simulink model "Missile"  (R2020a)
settings: Solver=VariableStepAuto  StartTime=0.0  StopTime=inf  RelTol=1e-3
InitFcn:
  | initKRPC
libraries: aerolibutil x2
settings Model: Creator=Administrator  LastModifiedBy=Administrator

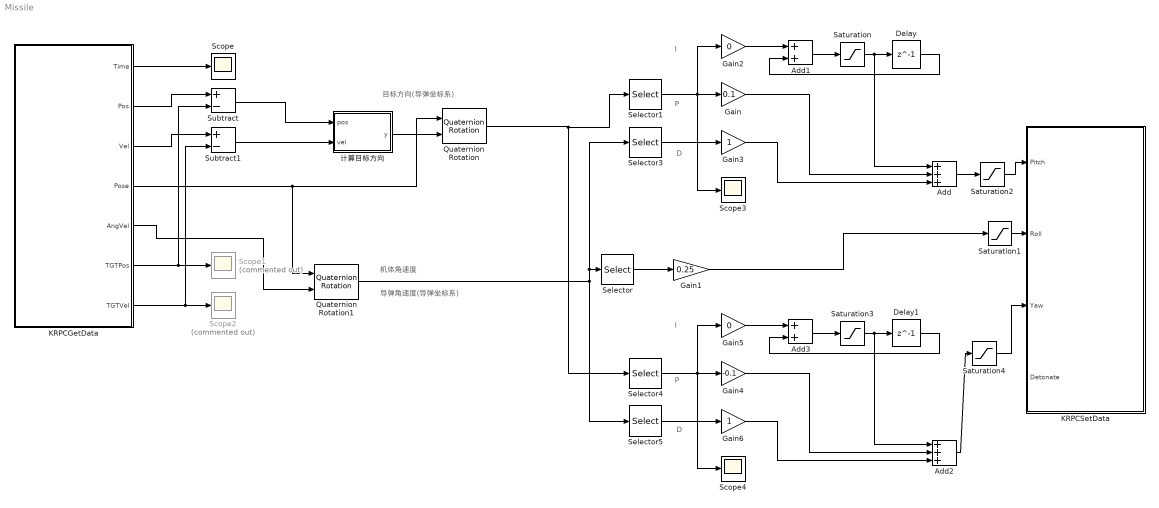
== system Missile ==
  note: D
  note: I
  note: P
  note: 目标方向(导弹坐标系)
  note: 机体角速度
  note: 导弹角速度(导弹坐标系)
  note: D
  note: P
  note: I
  Add : Sum  Inputs=+++
  Add1 : Sum
  Add2 : Sum  Inputs=+++
  Add3 : Sum
  Delay : Delay  DelayLength=1
  Delay1 : Delay  DelayLength=1
  Gain : Gain  Gain=0.1
  Gain1 : Gain  Gain=0.25
  Gain2 : Gain  Gain=0
  Gain3 : Gain
  Gain4 : Gain  Gain=-0.1
  Gain5 : Gain  Gain=0
  Gain6 : Gain
  KRPCGetData : MATLAB Function  TreatAsAtomicUnit=on
  KRPCSetData : MATLAB Function  TreatAsAtomicUnit=on
  Quaternion Rotation : aerolibutil/Quaternion Rotation
  Quaternion Rotation1 : aerolibutil/Quaternion Rotation
  Saturation : Saturate
  Saturation1 : Saturate  UpperLimit=1  LowerLimit=-1
  Saturation2 : Saturate  UpperLimit=1  LowerLimit=-1
  Saturation3 : Saturate
  Saturation4 : Saturate  UpperLimit=1  LowerLimit=-1
  Scope : Scope
  Scope1 : Scope  Commented=on
  Scope2 : Scope  Commented=on
  Scope3 : Scope
  Scope4 : Scope
  Selector : Selector  InputPortWidth=3  IndexOptions=Index vector (dialog)  Indices=2  OutputSizes=1
  Selector1 : Selector  InputPortWidth=3  IndexOptions=Index vector (dialog)  Indices=3  OutputSizes=1
  Selector3 : Selector  InputPortWidth=3  IndexOptions=Index vector (dialog)  Indices=1  OutputSizes=1
  Selector4 : Selector  InputPortWidth=3  IndexOptions=Index vector (dialog)  Indices=1  OutputSizes=1
  Selector5 : Selector  InputPortWidth=3  IndexOptions=Index vector (dialog)  Indices=3  OutputSizes=1
  Subtract : Sum  Inputs=+-
  Subtract1 : Sum  Inputs=+-
  计算目标方向 : MATLAB Function  TreatAsAtomicUnit=on
  wires:
  KRPCGetData/1(Time) -> Scope/1
  KRPCGetData/6(TGTPos) -> Subtract/2, Scope1/1
  KRPCGetData/7(TGTVel) -> Subtract1/2, Scope2/1
  KRPCGetData/4(Pose) -> Quaternion Rotation/1, Quaternion Rotation1/1
  KRPCGetData/5(AngVel) -> Quaternion Rotation1/2
  Quaternion Rotation1/1 -> Selector3/1, Selector/1, Selector5/1
  Selector/1 -> Gain1/1
  Saturation1/1 -> KRPCSetData/2(Roll)
  Gain1/1 -> Saturation1/1
  Selector1/1 -> Scope3/1, Gain2/1, Gain/1
  Gain/1 -> Add/2
  Add/1 -> Saturation2/1
  Saturation2/1 -> KRPCSetData/1(Pitch)
  Add1/1 -> Saturation/1
  Saturation/1 -> Add/1, Delay/1
  Delay/1 -> Add1/2
  Gain2/1 -> Add1/1
  Selector3/1 -> Gain3/1
  Gain3/1 -> Add/3
  Add3/1 -> Saturation3/1
  Selector4/1 -> Scope4/1, Gain5/1, Gain4/1
  Gain4/1 -> Add2/2
  Add2/1 -> Saturation4/1
  Gain6/1 -> Add2/3
  Saturation3/1 -> Add2/1, Delay1/1
  Gain5/1 -> Add3/1
  Delay1/1 -> Add3/2
  Selector5/1 -> Gain6/1
  Subtract/1 -> 计算目标方向/1(pos)
  Subtract1/1 -> 计算目标方向/2(vel)
  KRPCGetData/2(Pos) -> Subtract/1
  KRPCGetData/3(Vel) -> Subtract1/1
  计算目标方向/1(y) -> Quaternion Rotation/2
  Quaternion Rotation/1 -> Selector4/1, Selector1/1
  Saturation4/1 -> KRPCSetData/3(Yaw)

== matlab function Missile/KRPCSetData ==
  settings: updateMethod=DISCRETE  sampleTime=0.02
  data: Pitch input; Roll input; Yaw input; Detonate input
function KRPCSetData(Pitch,Roll,Yaw,Detonate)
coder.extrinsic('pushData');
pushData([Pitch,Roll,Yaw,Detonate]);

== matlab function Missile/KRPCGetData ==
  settings: updateMethod=DISCRETE  sampleTime=0.02
  data: Time output double size=1; Pos output double size=3; Vel output double size=3; Pose output double size=4; AngVel output double size=3; TGTPos output double size=3; TGTVel output double size=3
function [Time,Pos,Vel,Pose,AngVel,TGTPos,TGTVel] = KRPCGetData()
coder.extrinsic('gatherData');
data = NaN(20,1);
data(:) = gatherData();
Time = data(1);
Pos = data(2:4);
Vel = data(5:7);
Pose = data(8:11);
AngVel = data(12:14);
TGTPos = data(15:17);
TGTVel = data(18:20);

== matlab function Missile/计算目标方向 ==
  data: pos input; y output; vel input
function y = fcn(pos,vel)
pos = pos ./ sqrt(sum(pos.^2));
verr = vel - dot(pos,vel) .* pos;
if(sqrt(sum(verr.^2)) > 10)
    verr = verr .* 10./sqrt(sum(verr.^2));
end
y = verr + pos*10;
